simulink model "hw2_q4"  (R2022b)
settings: Solver=ode4  StartTime=0.0  StopTime=10.0  FixedStep=0.001  RelTol=1e-3
settings Model: Creator=gaura  LastModifiedBy=gaura

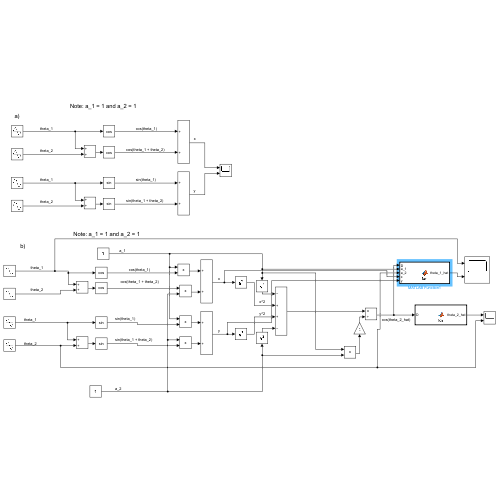
[thumbnail: Simulink's stored preview of the top-level diagram]
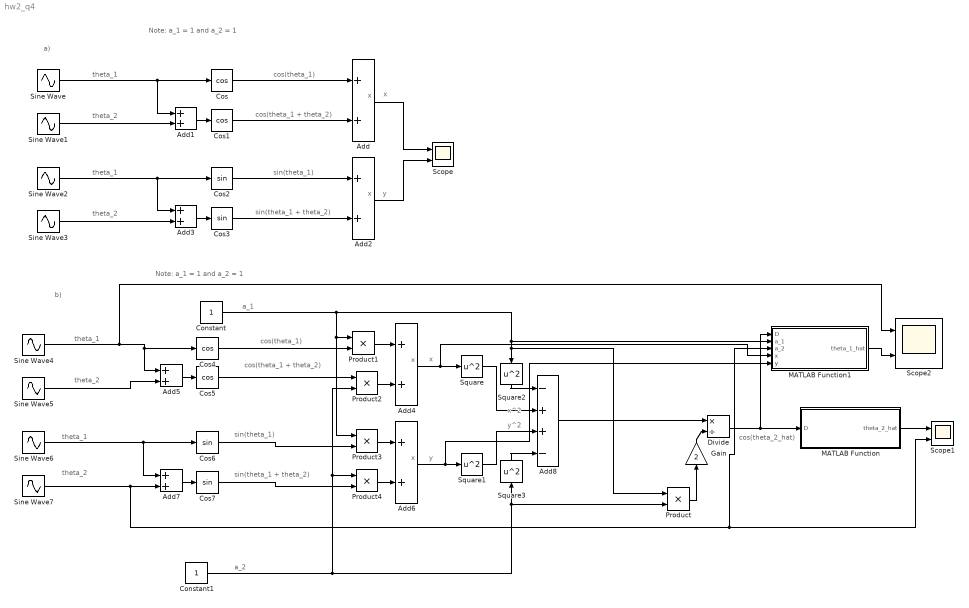
== system hw2_q4 ==
  note: a)
  note: cos(theta_2_hat)
  note: x^2
  note: y^2
  note: a_1
  note: y
  note: x
  note: y
  note: x
  note: Note: a_1 = 1 and a_2 = 1
  note: cos(theta_1)
  note: theta_1
  note: x
  note: theta_2
  note: cos(theta_1 + theta_2)
  note: x
  note: theta_2
  note: theta_1
  note: sin(theta_1)
  note: sin(theta_1 + theta_2)
  note: x
  note: sin(theta_1 + theta_2)
  note: theta_2
  note: theta_1
  note: theta_1
  note: sin(theta_1)
  note: cos(theta_1)
  note: theta_2
  note: x
  note: a_2
  note: cos(theta_1 + theta_2)
  note: b)
  note: Note: a_1 = 1 and a_2 = 1
  Add{,1..7} (8 alike) : Sum
  Add8 : Sum  Inputs=-++-
  Constant : Constant
  Constant1 : Constant
  Cos{,1,4..5} (4 alike) : Trigonometry  Operator=cos
  Cos{2..3,6..7} (4 alike) : Trigonometry
  Divide : Product  Inputs=*/
  Gain : Gain  Gain=2
  MATLAB Function : MATLAB Function  TreatAsAtomicUnit=on
  MATLAB Function1 : MATLAB Function  TreatAsAtomicUnit=on
  Product{,1..4} (5 alike) : Product
  Scope : Scope  NumInputPorts=2
  Scope1 : Scope  NumInputPorts=2
  Scope2 : Scope  NumInputPorts=2
  Sine Wave{,2,4,6} (4 alike) : Sin  SampleTime=0
  Sine Wave{1,3,5,7} (4 alike) : Sin  Frequency=5  SampleTime=0
  Square{,1..3} (4 alike) : Math  Operator=square
  wires:
  Add/1 -> Scope/1
  Sine Wave/1 -> Add1/1, Cos/1
  Cos/1 -> Add/1
  Cos1/1 -> Add/2
  Sine Wave1/1 -> Add1/2
  Add1/1 -> Cos1/1
  Add2/1 -> Scope/2
  Cos2/1 -> Add2/1
  Sine Wave3/1 -> Add3/2
  Sine Wave2/1 -> Add3/1, Cos2/1
  Cos3/1 -> Add2/2
  Add3/1 -> Cos3/1
  Add4/1 -> MATLAB Function1/4(x), Square/1
  Sine Wave7/1 -> MATLAB Function1/3(a_2), Scope1/2, Add7/2
  Sine Wave6/1 -> Add7/1, Cos6/1
  Add7/1 -> Cos7/1
  Add6/1 -> MATLAB Function1/5(y), Square1/1
  Cos4/1 -> Product1/2
  Sine Wave5/1 -> Add5/2
  Sine Wave4/1 -> Scope2/1, Add5/1, Cos4/1
  Add5/1 -> Cos5/1
  Constant/1 -> Product3/1, Product1/1, MATLAB Function1/2(a_1), Product/1, Square2/1
  Square/1 -> Add8/2
  Constant1/1 -> Product2/2, Product4/1, Product/2, Square3/1
  Square1/1 -> Add8/3
  Add8/1 -> Divide/1
  Product/1 -> Gain/1
  Divide/1 -> MATLAB Function1/1(D), MATLAB Function/1(D)
  MATLAB Function/1(theta_2_hat) -> Scope1/1
  Gain/1 -> Divide/2
  Square2/1 -> Add8/1
  Square3/1 -> Add8/4
  Product1/1 -> Add4/1
  Cos6/1 -> Product3/2
  Product3/1 -> Add6/1
  Cos7/1 -> Product4/2
  Cos5/1 -> Product2/1
  Product2/1 -> Add4/2
  Product4/1 -> Add6/2
  MATLAB Function1/1(theta_1_hat) -> Scope2/2

== matlab function hw2_q4/MATLAB Function1 ==
  data: D input; theta_1_hat output; a_1 input; a_2 input; x input; y input
function theta_1_hat = fcn(D, a_1, a_2, x, y)

% numerator = y*(a_1 + a_2 * D) - x*a_2*sqrt(1-D.^2);
% denominator = x*(a_1 + a_2*D + y*a_2*sqrt(1-D.^2));

% theta_1_hat = atan(numerator/denominator);
k1 = a_1 + a_2.*D;
k2 = a_2*sqrt(1-D.^2);

theta_1_hat = atan2(y,x) - atan2(k2,k1);

== matlab function hw2_q4/MATLAB Function ==
  data: D input; theta_2_hat output
function theta_2_hat = fcn(D)

% also works
% theta_2_hat = atan(sqrt(1-(D^2))/D);

theta_2_hat = atan(sqrt(1-(D^2))/D);
